simulink model "DynamixelLibrary_Prototyping"  (R2020a)
settings: Solver=FixedStepAuto  StartTime=0.0  StopTime=30  FixedStep=0.05  RelTol=1e-3  EnableMultiTasking=on
undefined symbols (not defined in the file or in its folder): DiscIntNeverNeededParam
libraries: simulink x3
settings Model: SimulationMode=external  Creator=AlexC  LastModifiedBy=SPOT
settings SolverCC: PositivePriorityOrder=on
settings DataIOCC: ReturnWorkspaceOutputs=off
settings OptimizationCC: PassReuseOutputArgsThreshold=0  MaxStackSize=64  EfficientTunableParamExpr=on
settings DebuggingCC: ParameterTunabilityLossMsg=error  ArithmeticOperatorsInVariantConditions=warning
settings HardwareCC: ProdBitPerPointer=32  ProdBitPerSizeT=32  ProdBitPerPtrDiffT=32  ProdLargestAtomicInteger=Long  ProdLargestAtomicFloat=Double  ProdWordSize=32  ProdHWDeviceType=ARM Compatible->ARM Cortex
settings SFSimCC: SimUseLocalCustomCode=off  MATLABDynamicMemAlloc=off  CustomCodeUndefinedFunction=UseInterfaceOnly
settings RTWCC: SystemTargetFile=ert.tlc  HardwareBoard=Raspberry Pi  TemplateMakefile=ert_default_tmf  RTWUseLocalCustomCode=off  Toolchain=GNU GCC Raspberry Pi  BuildConfiguration=Specify  TargetLang=C++
settings CodeAppCC: ForceParamTrailComments=on  OperatorAnnotations=on
settings ERTTargetCC: CodeReplacementLibrary=GCC ARM Cortex-A8  ERTCustomFileBanners=off  SupportContinuousTime=on  SupportNonInlinedSFcns=on  RemoveResetFunc=off  SupportVariableSizeSignals=on  ModelStepFunctionPrototypeControlCompliant=off  RootIOFormat=Structure reference

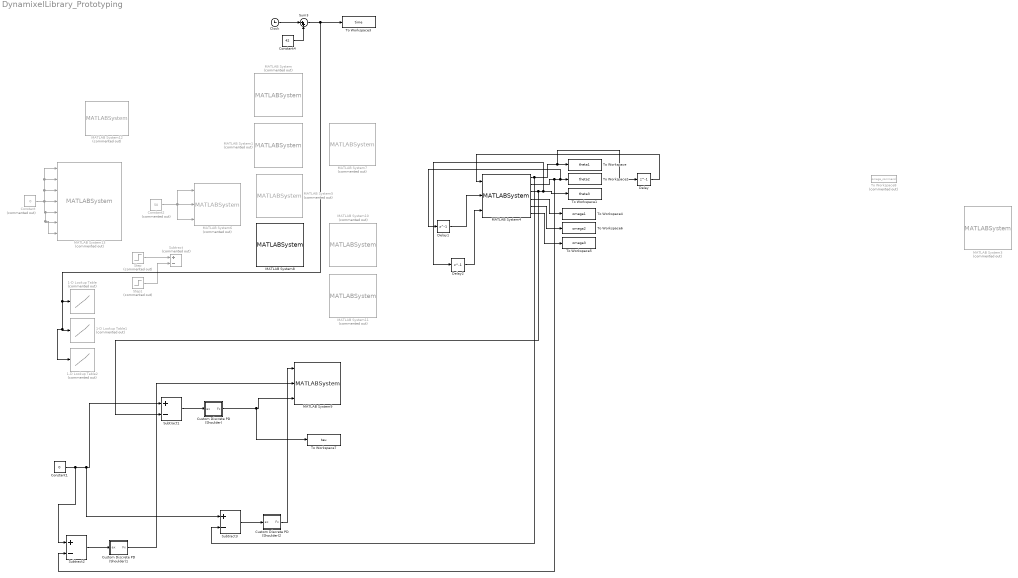
== system DynamixelLibrary_Prototyping ==
  1-D Lookup Table : Lookup_n-D  Commented=on  NumberOfTableDimensions=1  BreakpointsForDimension1=|  Table=|  InternalRulePriority=Speed  RndMeth=Simplest  InputSameDT=on
      BreakpointsForDimension1=|
      | [42
      | 42.01112133
      | 42.03727126
      | 42.07834039
      | 42.13428459
      | 42.20504754
      | 42.29055854
      | 42.39073228
      | 42.5054689
      | 42.63465399
      | 42.77815879
      | 42.93584024
      | 43.10754115
      | 43.29309037
      | 43.49230294
      | 43.70498028
      | 43.93091039
      | 44.16986804
      | 44.42161506
      | 44.68590048
      | 44.96246087
      | 45.25102053
      | 45.55129184
      | 45.86297547
      | 46.18576072
      | 46.51932585
      | 46.86333834
      | 47.21745527
      | 47.58132366
      | 47.95458079
      | 48.33685459
      | 48.727764
      | 49.12691936
      | 49.53392277
      | 49.94836853
      | 50.36984352
      | 50.79792758
      | 51.23219401
      | 51.67220991
      | 52.11753667
      | 52.56773038
      | 53.02234226
      | 53.48091917
      | 53.94300397
      | 54.40813605
      | 54.87585175
      | 55.34568486
      | 55.81716702
      | 56.28982825
      | 56.7631974
      | 57.2368026
      | 57.71017175
      | 58.18283298
      | 58.65431514
      | 59.12414825
      | 59.59186395
      | 60.05699603
      | 60.51908083
      | 60.97765774
      | 61.43226962
      | 61.88246333
      | 62.32779009
      | 62.76780599
      | 63.20207242
      | 63.63015648
      | 64.05163147
      | 64.46607723
      | 64.87308064
      | 65.272236
      | 65.66314541
      | 66.04541921
      | 66.41867634
      | 66.78254473
      | 67.13666166
      | 67.48067415
      | 67.81423928
      | 68.13702453
      | 68.44870816
      | 68.74897947
      | 69.03753913
      | 69.31409952
      | 69.57838494
      | 69.83013196
      | 70.06908961
      | 70.29501972
      | 70.50769706
      | 70.70690963
      | 70.89245885
      | 71.06415976
      | 71.22184121
      | 71.36534601
      | 71.4945311
      | 71.60926772
      | 71.70944146
      | 71.79495246
      | 71.86571541
      | 71.92165961
      | 71.96272874
      | 71.98887867
      | 72
      | ]
      Table=|
      | [1.570796327
      | 1.570792957
      | 1.570647694
      | 1.56961565
      | 1.567632601
      | 1.56219496
      | 1.557494298
      | 1.549269077
      | 1.544187815
      | 1.533149542
      | 1.522693414
      | 1.496131515
      | 1.446175572
      | 1.373291416
      | 1.270392573
      | 1.167493418
      | 1.052460989
      | 0.935207834
      | 0.807889258
      | 0.677163853
      | 0.538528963
      | 0.394913096
      | 0.249656169
      | 0.099916299
      | -0.053813644
      | -0.205103655
      | -0.380299244
      | -0.546735993
      | -0.717860815
      | -0.811444171
      | -0.923417052
      | -0.9559831
      | -0.833382367
      | -0.653115778
      | -0.440627342
      | -0.233135617
      | -0.016770488
      | 0.198541763
      | 0.420037648
      | 0.64133109
      | 0.8678487
      | 1.093144441
      | 1.326954733
      | 1.513077918
      | 1.568710242
      | 1.570730531
      | 1.567250769
      | 1.570752371
      | 1.57074092
      | 1.549011834
      | 1.401751602
      | 1.165146113
      | 1.0076873
      | 0.810904438
      | 0.65519077
      | 0.460795111
      | 0.26479445
      | 0.068785172
      | -0.154928236
      | -0.361424338
      | -0.588740331
      | -0.797757514
      | -1.025114417
      | -1.236311075
      | -1.435945334
      | -1.511406602
      | -1.466017975
      | -1.310813705
      | -1.105992736
      | -0.913718388
      | -0.722685301
      | -0.536202121
      | -0.354350457
      | -0.177037457
      | -0.005416103
      | 0.161859666
      | 0.322652337
      | 0.479244088
      | 0.627815916
      | 0.771700562
      | 0.909552257
      | 1.042365309
      | 1.164760086
      | 1.265366299
      | 1.329745445
      | 1.358265779
      | 1.355564401
      | 1.328554047
      | 1.279612684
      | 1.24723853
      | 1.197192467
      | 1.141005155
      | 1.106426692
      | 1.08119376
      | 1.067581158
      | 1.058578831
      | 1.055001377
      | 1.05322972
      | 1.052803704
      | 1.052721605
      | ]
  1-D Lookup Table1 : Lookup_n-D  Commented=on  NumberOfTableDimensions=1  BreakpointsForDimension1=|  Table=|  InternalRulePriority=Speed  RndMeth=Simplest  InputSameDT=on
      BreakpointsForDimension1=|
      | [42
      | 42.01112133
      | 42.03727126
      | 42.07834039
      | 42.13428459
      | 42.20504754
      | 42.29055854
      | 42.39073228
      | 42.5054689
      | 42.63465399
      | 42.77815879
      | 42.93584024
      | 43.10754115
      | 43.29309037
      | 43.49230294
      | 43.70498028
      | 43.93091039
      | 44.16986804
      | 44.42161506
      | 44.68590048
      | 44.96246087
      | 45.25102053
      | 45.55129184
      | 45.86297547
      | 46.18576072
      | 46.51932585
      | 46.86333834
      | 47.21745527
      | 47.58132366
      | 47.95458079
      | 48.33685459
      | 48.727764
      | 49.12691936
      | 49.53392277
      | 49.94836853
      | 50.36984352
      | 50.79792758
      | 51.23219401
      | 51.67220991
      | 52.11753667
      | 52.56773038
      | 53.02234226
      | 53.48091917
      | 53.94300397
      | 54.40813605
      | 54.87585175
      | 55.34568486
      | 55.81716702
      | 56.28982825
      | 56.7631974
      | 57.2368026
      | 57.71017175
      | 58.18283298
      | 58.65431514
      | 59.12414825
      | 59.59186395
      | 60.05699603
      | 60.51908083
      | 60.97765774
      | 61.43226962
      | 61.88246333
      | 62.32779009
      | 62.76780599
      | 63.20207242
      | 63.63015648
      | 64.05163147
      | 64.46607723
      | 64.87308064
      | 65.272236
      | 65.66314541
      | 66.04541921
      | 66.41867634
      | 66.78254473
      | 67.13666166
      | 67.48067415
      | 67.81423928
      | 68.13702453
      | 68.44870816
      | 68.74897947
      | 69.03753913
      | 69.31409952
      | 69.57838494
      | 69.83013196
      | 70.06908961
      | 70.29501972
      | 70.50769706
      | 70.70690963
      | 70.89245885
      | 71.06415976
      | 71.22184121
      | 71.36534601
      | 71.4945311
      | 71.60926772
      | 71.70944146
      | 71.79495246
      | 71.86571541
      | 71.92165961
      | 71.96272874
      | 71.98887867
      | 72
      | ]
      Table=|
      | [1.57079632679490
      | 1.57079662136271
      | 1.57035858393418
      | 1.56955473957150
      | 1.56795883023701
      | 1.56855196252543
      | 1.56956191136717
      | 1.57072970527338
      | 1.57079005485722
      | 1.56948791223666
      | 1.55119006552306
      | 1.55836585845583
      | 1.57077777185491
      | 1.57077149370545
      | 1.57076310797240
      | 1.57036928804412
      | 1.57074947684855
      | 1.56898331366692
      | 1.57073740451593
      | 1.56257826917437
      | 1.57072974696569
      | 1.56230742665956
      | 1.57073312881541
      | 1.56360724537446
      | 1.57075185491036
      | 1.56920954766940
      | 1.57077382899638
      | 1.54477346684241
      | 1.38400507014983
      | 1.23109269186081
      | 1.02321737126326
      | 0.866665055111140
      | 0.663320579242585
      | 0.523334911886864
      | 0.348534652658928
      | 0.228481728516264
      | 0.156644623807384
      | 0.0854385589397119
      | 0.0684187356026291
      | -0.0143597952556130
      | -0.0517524216410004
      | -0.0928804549026143
      | -0.215704480084781
      | -0.422252680325216
      | -0.607845118006062
      | -0.846263996013364
      | -1.04958098308095
      | -1.27739473865326
      | -1.42310649047080
      | -1.57075277736191
      | -1.57072459354704
      | -1.57072993276777
      | -1.54331811766860
      | -1.57073414073308
      | -1.55931623516956
      | -1.57073842553777
      | -1.57072399077284
      | -1.57072720156105
      | -1.57071264380253
      | -1.56934197452670
      | -1.57070564382063
      | -1.56141817042798
      | -1.57070830688086
      | -1.49469854852628
      | -1.31259934378585
      | -1.11020895684375
      | -0.916078821647610
      | -0.731793274192232
      | -0.573229556030265
      | -0.475634259727501
      | -0.252113034776861
      | -0.175932768714599
      | -0.117451385657779
      | -0.113075584941122
      | -0.108548532723191
      | -0.120323450723243
      | -0.116071199535664
      | -0.122092030089114
      | -0.179069682787195
      | -0.187679506880811
      | -0.283142131452161
      | -0.409036068532655
      | -0.536944980678811
      | -0.655297933993903
      | -0.768540738868273
      | -0.875433002578302
      | -0.973536605110186
      | -1.06911393555782
      | -1.14791786909907
      | -1.22902449271238
      | -1.27006052589809
      | -1.28669314276116
      | -1.31617501989999
      | -1.33099075176741
      | -1.34662299508091
      | -1.35249457213426
      | -1.35797341773929
      | -1.35939252934314
      | -1.35990006404006
      | -1.35985448160842]
  1-D Lookup Table2 : Lookup_n-D  Commented=on  NumberOfTableDimensions=1  BreakpointsForDimension1=|  Table=|  InternalRulePriority=Speed  RndMeth=Simplest  InputSameDT=on
      BreakpointsForDimension1=|
      | [42
      | 42.01112133
      | 42.03727126
      | 42.07834039
      | 42.13428459
      | 42.20504754
      | 42.29055854
      | 42.39073228
      | 42.5054689
      | 42.63465399
      | 42.77815879
      | 42.93584024
      | 43.10754115
      | 43.29309037
      | 43.49230294
      | 43.70498028
      | 43.93091039
      | 44.16986804
      | 44.42161506
      | 44.68590048
      | 44.96246087
      | 45.25102053
      | 45.55129184
      | 45.86297547
      | 46.18576072
      | 46.51932585
      | 46.86333834
      | 47.21745527
      | 47.58132366
      | 47.95458079
      | 48.33685459
      | 48.727764
      | 49.12691936
      | 49.53392277
      | 49.94836853
      | 50.36984352
      | 50.79792758
      | 51.23219401
      | 51.67220991
      | 52.11753667
      | 52.56773038
      | 53.02234226
      | 53.48091917
      | 53.94300397
      | 54.40813605
      | 54.87585175
      | 55.34568486
      | 55.81716702
      | 56.28982825
      | 56.7631974
      | 57.2368026
      | 57.71017175
      | 58.18283298
      | 58.65431514
      | 59.12414825
      | 59.59186395
      | 60.05699603
      | 60.51908083
      | 60.97765774
      | 61.43226962
      | 61.88246333
      | 62.32779009
      | 62.76780599
      | 63.20207242
      | 63.63015648
      | 64.05163147
      | 64.46607723
      | 64.87308064
      | 65.272236
      | 65.66314541
      | 66.04541921
      | 66.41867634
      | 66.78254473
      | 67.13666166
      | 67.48067415
      | 67.81423928
      | 68.13702453
      | 68.44870816
      | 68.74897947
      | 69.03753913
      | 69.31409952
      | 69.57838494
      | 69.83013196
      | 70.06908961
      | 70.29501972
      | 70.50769706
      | 70.70690963
      | 70.89245885
      | 71.06415976
      | 71.22184121
      | 71.36534601
      | 71.4945311
      | 71.60926772
      | 71.70944146
      | 71.79495246
      | 71.86571541
      | 71.92165961
      | 71.96272874
      | 71.98887867
      | 72
      | ]
      Table=|
      | [-1.10360555189321e-17
      | -0.000682555954124297
      | -0.000504375242443253
      | 0.00336297359381415
      | 0.0137095670724727
      | 0.0252677971790659
      | 0.0446557220510096
      | 0.0672113326003172
      | 0.0999781977666613
      | 0.137287456967193
      | 0.189071248486376
      | 0.272294508037825
      | 0.355665679231944
      | 0.446845913729827
      | 0.544137284526667
      | 0.639346413276106
      | 0.732541458867562
      | 0.808938354869002
      | 0.855848674103189
      | 0.891616122311551
      | 0.876064789878543
      | 0.835218274860764
      | 0.735847487773707
      | 0.623237833236767
      | 0.450912596118759
      | 0.313068707480842
      | 0.118982751928026
      | -0.0346963999777990
      | -0.244244268013732
      | -0.386045753956551
      | -0.607135995230889
      | -0.645065479955685
      | -0.658232101032023
      | -0.707283001569499
      | -0.727739337943063
      | -0.773334139757485
      | -0.790813868197939
      | -0.829315581367480
      | -0.831591865361474
      | -0.895741116707505
      | -0.917692198886409
      | -0.966835773186509
      | -1.05732301030663
      | -1.15418729750044
      | -1.28905944926691
      | -1.41505461173534
      | -1.40486598987903
      | -1.38850533888304
      | -1.31148648974968
      | -1.22739644537344
      | -1.09679708257291
      | -1.01375741649069
      | -0.900389419892854
      | -0.817697106109663
      | -0.706296706872995
      | -0.627649901158471
      | -0.522783214749143
      | -0.449254069405809
      | -0.350308226521183
      | -0.271181857633944
      | -0.185730374564875
      | -0.134238582279295
      | -0.0589333568892688
      | -0.0193632216828676
      | 0.0500980441953301
      | 0.0783818433368992
      | 0.203392718385905
      | 0.287418813233287
      | 0.286916152215522
      | 0.228277773431529
      | 0.205391483508272
      | 0.153166933412198
      | 4.01249706205260e-05
      | -0.106583281044124
      | -0.214939176631723
      | -0.275105513577021
      | -0.328996825397653
      | -0.353637536054736
      | -0.366278937268333
      | -0.349072653017436
      | -0.324125317636826
      | -0.291582405014021
      | -0.240949835499918
      | -0.195848531903513
      | -0.143488080387155
      | -0.0988801304986467
      | -0.0443831356850743
      | 0.00807376276159867
      | 0.0766461923527033
      | 0.116804310925055
      | 0.159885004199221
      | 0.212747759359235
      | 0.240304582731963
      | 0.265011768867661
      | 0.280740585503698
      | 0.294154580752225
      | 0.300980006322197
      | 0.305531467486406
      | 0.306822115333088
      | 0.307132876918720]
  Clock : Clock
  Constant : Constant  Commented=on  Value=0
  Constant1 : Constant  Value=0
  Constant2 : Constant  Commented=on  Value=50
  Constant4 : Constant  Value=42
  Custom Discrete PD (Shoulder) : Subsystem
  Custom Discrete PD (Shoulder)1 : Subsystem
  Custom Discrete PD (Shoulder)2 : Subsystem
  Delay : Delay  DelayLength=1
  Delay1 : Delay  DelayLength=1
  Delay2 : Delay  DelayLength=1
  MATLAB System : MATLABSystem  Commented=on  System=InitializeForPosition  P_GAIN=400  I_GAIN=0  D_GAIN=200  MAX_POSITION=3072  MIN_POSITION=1024  MOVE_TIME=500
      mask Type: InitializeForPosition
      mask Display: disp('InitializeForPosition');
  MATLAB System1 : MATLABSystem  Commented=on  System=InitializeForSpeed  P_GAIN=100  I_GAIN=1920  VELOCITY_LIMIT=22
      mask Type: InitializeForSpeed
      mask Display: disp('InitializeForSpeed');
  MATLAB System10 : MATLABSystem  Commented=on  System=InitializeForSpecial  CURRENT_LIMIT=850  P_GAIN=400  I_GAIN=0  D_GAIN=200  MAX_POSITION=3072  MIN_POSITION=1024  VELOCITY_LIMIT=0
      mask Type: InitializeForSpecial
      mask Display: disp('InitializeForSpecial');
  MATLAB System11 : MATLABSystem  Commented=on  System=MoveArm_Special
      mask Type: MoveArm_Special
      mask Display:
      | disp('MoveArm_Special');
      | port_label('input',1,'u1');
      | port_label('input',2,'u2');
      | port_label('input',3,'u3');
  MATLAB System12 : MATLABSystem  Commented=on  System=InitializeForArmGripper  P_GAIN_ARM=400  I_GAIN_ARM=0  D_GAIN_ARM=200  P_GAIN_PROX=400  I_GAIN_PROX=0  D_GAIN_PROX=200  P_GAIN_DIST=400  I_GAIN_DIST=0  D_GAIN_DIST=200  MAX_POSITION_ARM=3072  MIN_POSITION_ARM=1024  MAX_POSITION_PROX=3072  MIN_POSITION_PROX=1024  MAX_POSITION_DIST=3072  MIN_POSITION_DIST=1024  VELOCITY_LIMIT_ARM=0  VELOCITY_LIMIT_GRIP=0  MAX_CURRENT_GRIP=1000
      mask Type: InitializeForArmGripper
      mask Display: disp('InitializeForArmGripper');
  MATLAB System13 : MATLABSystem  Commented=on  System=MoveArmGripper_Position
      mask Type: MoveArmGripper_Position
      mask Display:
      | disp('MoveArmGripper_Position');
      | port_label('input',1,'u1');
      | port_label('input',2,'u2');
      | port_label('input',3,'u3');
      | port_label('input',4,'uL1');
      | port_label('input',5,'uR1');
      | port_label('input',6,'uL2');
      | port_label('input',7,'uR2');
  MATLAB System3 : MATLABSystem  Commented=on  System=MoveArm_Speed
      mask Type: MoveArm_Speed
      mask Display:
      | disp('MoveArm_Speed');
      | port_label('input',1,'u1');
      | port_label('input',2,'u2');
      | port_label('input',3,'u3');
      | port_label('input',4,'accel_time');
  MATLAB System4 : MATLABSystem  System=ReadArm_Position_Rates  SampleTime=0.05
      mask Type: ReadArm_Position_Rates
      mask Display:
      | disp('ReadArm_Position_Rates');
      | port_label('input',1,'u1');
      | port_label('input',2,'u2');
      | port_label('input',3,'u3');
      | port_label('output',1,'theta1');
      | port_label('output',2,'theta2');
      | port_label('output',3,'theta3');
      | port_label('output',4,'omega1');
      | port_label('output',5,'omega2');
      | port_label('output',6,'omega3');
  MATLAB System5 : MATLABSystem  Commented=on  System=InitializeForPWM  PWM_LIMIT=885
      mask Type: InitializeForPWM
      mask Display: disp('InitializeForPWM');
  MATLAB System6 : MATLABSystem  Commented=on  System=MoveArm_PWM
      mask Type: MoveArm_PWM
      mask Display:
      | disp('MoveArm_PWM');
      | port_label('input',1,'u1');
      | port_label('input',2,'u2');
      | port_label('input',3,'u3');
  MATLAB System7 : MATLABSystem  Commented=on  System=ReadArm_Load  SampleTime=0.1
      mask Type: ReadArm_Load
      mask Display:
      | disp('ReadArm_Load');
      | port_label('output',1,'y1');
      | port_label('output',2,'y2');
      | port_label('output',3,'y3');
  MATLAB System8 : MATLABSystem  System=InitializeForTorque  CURRENT_LIMIT=2000
      mask Type: InitializeForTorque
      mask Display: disp('InitializeForTorque');
  MATLAB System9 : MATLABSystem  System=MoveArm_Torque
      mask Type: MoveArm_Torque
      mask Display:
      | disp('MoveArm_Torque');
      | port_label('input',1,'u1');
      | port_label('input',2,'u2');
      | port_label('input',3,'u3');
  Step : Step  Commented=on  Time=5  After=30  SampleTime=0
  Step1 : Step  Commented=on  Time=6  After=30  SampleTime=0
  Subtract : Sum  Commented=on  Inputs=+-
  Subtract1 : Sum  Inputs=+-
  Subtract2 : Sum  Inputs=+-
  Subtract3 : Sum  Inputs=+-
  Sum3 : Sum  Inputs=|++
  To Workspace : ToWorkspace  VariableName=theta1  SampleTime=-1
      settings: Save2DSignal=2-D array (concatenate along first dimension)
  To Workspace1 : ToWorkspace  VariableName=theta3  SampleTime=-1
      settings: Save2DSignal=2-D array (concatenate along first dimension)
  To Workspace2 : ToWorkspace  VariableName=theta2  SampleTime=-1
      settings: Save2DSignal=2-D array (concatenate along first dimension)
  To Workspace3 : ToWorkspace  VariableName=time  SampleTime=-1
  To Workspace4 : ToWorkspace  VariableName=omega1  SampleTime=-1
      settings: Save2DSignal=2-D array (concatenate along first dimension)
  To Workspace5 : ToWorkspace  VariableName=omega3  SampleTime=-1
      settings: Save2DSignal=2-D array (concatenate along first dimension)
  To Workspace6 : ToWorkspace  VariableName=omega2  SampleTime=-1
      settings: Save2DSignal=2-D array (concatenate along first dimension)
  To Workspace7 : ToWorkspace  VariableName=tau  SampleTime=-1
      settings: Save2DSignal=2-D array (concatenate along first dimension)
  To Workspace8 : ToWorkspace  Commented=on  VariableName=omega_command  SampleTime=-1
  wires:
  Constant2/1 -> MATLAB System6/3, MATLAB System6/1, MATLAB System6/2
  Step/1 -> Subtract/1
  Step1/1 -> Subtract/2
  Constant/1 -> MATLAB System13/7, MATLAB System13/6, MATLAB System13/5, MATLAB System13/3, MATLAB System13/2, MATLAB System13/1, MATLAB System13/4
  MATLAB System4/2 -> Subtract2/2, Delay1/1, To Workspace2/1
  MATLAB System4/3 -> Subtract1/2, Delay2/1, To Workspace1/1
  MATLAB System4/4 -> To Workspace4/1
  MATLAB System4/5 -> To Workspace6/1
  MATLAB System4/6 -> To Workspace5/1
  ? -> To Workspace8/1, MATLAB System3/1
  ? -> MATLAB System3/2
  ? -> MATLAB System3/3
  Clock/1 -> Sum3/1
  MATLAB System4/1 -> Delay/1, To Workspace/1, Subtract3/2
  Delay/1 -> MATLAB System4/1
  Delay1/1 -> MATLAB System4/2
  Delay2/1 -> MATLAB System4/3
  Subtract1/1 -> Custom Discrete PD (Shoulder)/1(ex)
  Custom Discrete PD (Shoulder)/1(Fx) -> To Workspace7/1, MATLAB System9/3
  Subtract2/1 -> Custom Discrete PD (Shoulder)1/1(ex)
  Custom Discrete PD (Shoulder)1/1(Fx) -> MATLAB System9/2
  Subtract3/1 -> Custom Discrete PD (Shoulder)2/1(ex)
  Custom Discrete PD (Shoulder)2/1(Fx) -> MATLAB System9/1
  Constant4/1 -> Sum3/2
  Sum3/1 -> 1-D Lookup Table2/1, 1-D Lookup Table1/1, 1-D Lookup Table/1, To Workspace3/1
  Constant1/1 -> Subtract2/1, Subtract3/1, Subtract1/1

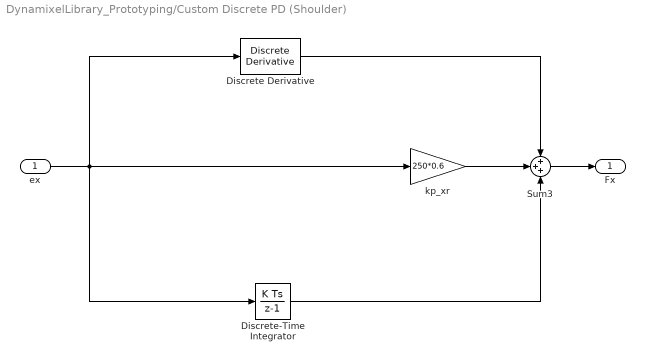
== system DynamixelLibrary_Prototyping/Custom Discrete PD (Shoulder) ==
  ex : Inport
  Discrete Derivative : simulink/Discrete/Discrete Derivative  gainval=0  ICPrevScaledInput=0.0  OutMin=[]  OutMax=[]  OutDataType=fixdt(1, 16)  OutScaling=2^-10  DoSatur=off
  Discrete-Time Integrator : DiscreteIntegrator  gainval=100  SampleTime=-1  ICPrevOutput=DiscIntNeverNeededParam  ICPrevScaledInput=DiscIntNeverNeededParam
  Sum3 : Sum  Inputs=+++
  kp_xr : Gain  Gain=250*0.6
  Fx : Outport  VectorParamsAs1DForOutWhenUnconnected=off
  wires:
  Discrete Derivative/1 -> Sum3/1
  ex/1 -> Discrete-Time Integrator/1, kp_xr/1, Discrete Derivative/1
  kp_xr/1 -> Sum3/2
  Sum3/1 -> Fx/1
  Discrete-Time Integrator/1 -> Sum3/3

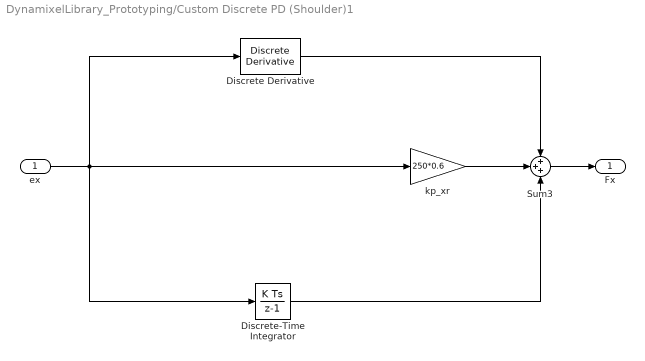
== system DynamixelLibrary_Prototyping/Custom Discrete PD (Shoulder)1 ==
  ex : Inport
  Discrete Derivative : simulink/Discrete/Discrete Derivative  gainval=0  ICPrevScaledInput=0.0  OutMin=[]  OutMax=[]  OutDataType=fixdt(1, 16)  OutScaling=2^-10  DoSatur=off
  Discrete-Time Integrator : DiscreteIntegrator  gainval=100  SampleTime=-1  ICPrevOutput=DiscIntNeverNeededParam  ICPrevScaledInput=DiscIntNeverNeededParam
  Sum3 : Sum  Inputs=+++
  kp_xr : Gain  Gain=250*0.6
  Fx : Outport  VectorParamsAs1DForOutWhenUnconnected=off
  wires:
  Discrete Derivative/1 -> Sum3/1
  ex/1 -> Discrete-Time Integrator/1, kp_xr/1, Discrete Derivative/1
  kp_xr/1 -> Sum3/2
  Sum3/1 -> Fx/1
  Discrete-Time Integrator/1 -> Sum3/3

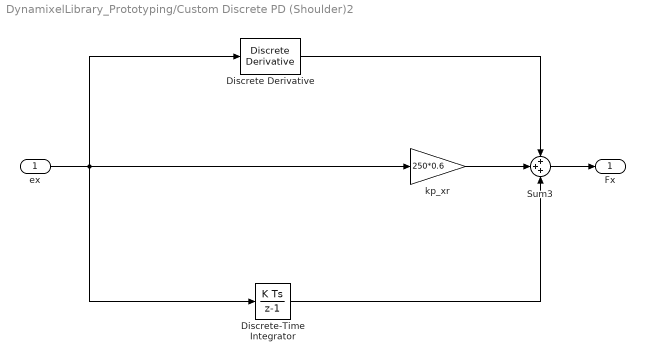
== system DynamixelLibrary_Prototyping/Custom Discrete PD (Shoulder)2 ==
  ex : Inport
  Discrete Derivative : simulink/Discrete/Discrete Derivative  gainval=50  ICPrevScaledInput=0.0  OutMin=[]  OutMax=[]  OutDataType=fixdt(1, 16)  OutScaling=2^-10  DoSatur=off
  Discrete-Time Integrator : DiscreteIntegrator  gainval=100  SampleTime=-1  ICPrevOutput=DiscIntNeverNeededParam  ICPrevScaledInput=DiscIntNeverNeededParam
  Sum3 : Sum  Inputs=+++
  kp_xr : Gain  Gain=250*0.6
  Fx : Outport  VectorParamsAs1DForOutWhenUnconnected=off
  wires:
  Discrete Derivative/1 -> Sum3/1
  ex/1 -> Discrete-Time Integrator/1, kp_xr/1, Discrete Derivative/1
  kp_xr/1 -> Sum3/2
  Sum3/1 -> Fx/1
  Discrete-Time Integrator/1 -> Sum3/3
